simulink model "quadcopter_model"  (R2021a)
settings: Solver=VariableStepAuto  StartTime=0.0  StopTime=500  RelTol=1e-3
values from neighbouring files (symbols this model uses):
  additive_noise = 0    [variables.m]
  initialCondition = [x0 vx0 y0 vy0 z0 vz0 phi0 p0 theta0 q0 psi0 r0]    [variables.m]
  param = [m;Ix;Iy;Iz;l;g]    [variables.m]
libraries: dspsrcs4 x1
settings Model: Creator=fiori  LastModifiedBy=fiori
settings SolverCC: AlgebraicLoopSolver=TrustRegion
settings DebuggingCC: SFMachineParentedDataDiag=warning

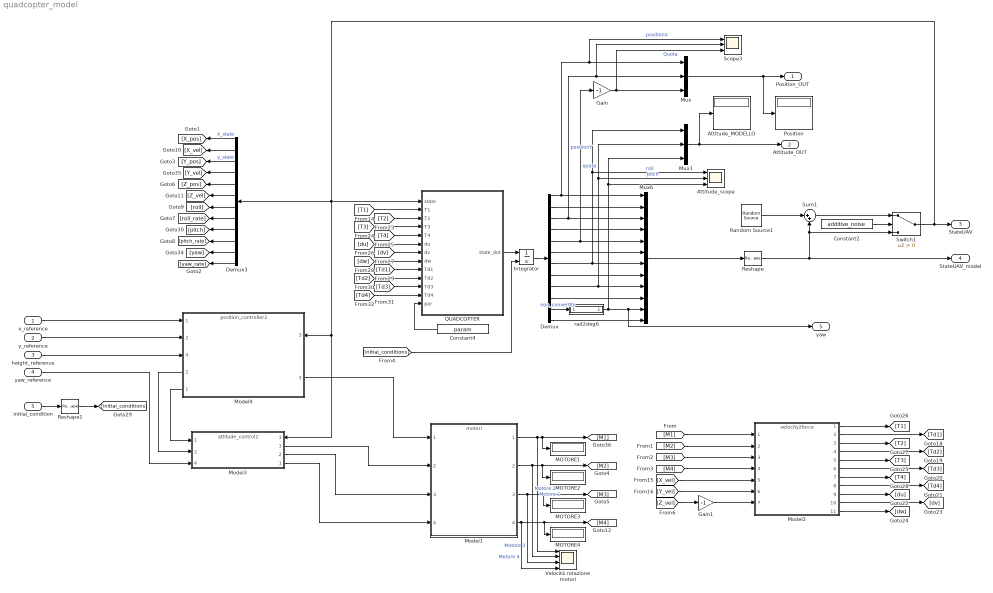
== system quadcopter_model ==
  x_reference : Inport
  y_reference : Inport  Port=2
  height_reference : Inport  Port=3
  yaw_reference : Inport  Port=4
  initial_condition : Inport  Port=5
  Attitude_MODELLO : Display
  Attitude_scope : Scope  NumInputPorts=3
  Constant2 : Constant  Value=additive_noise
  Constant4 : Constant  Value=param
  Demux : Demux  Outputs=12
  Demux3 : Demux  Outputs=12
  Gain : Gain  Gain=-1
  Gain1 : Gain  Gain=-1
  Integrator : Integrator  InitialConditionSource=external  InitialCondition=initialCondition
  MOTORE{1..4} (4 alike) : Display
  Model1 : ModelReference  ModelNameDialog=motori.slx  SimulationMode=Normal  ModelReferenceVersion=1.1
  Model2 : ModelReference  ModelNameDialog=velocity2force.slx  SimulationMode=Normal  ModelReferenceVersion=1.6
  Model3 : ModelReference  ModelNameDialog=attitude_control2.slx  SimulationMode=Normal  ModelReferenceVersion=2.5
      settings: PortSchema="{\"entries\":[{\"content\":{\"sides\":[{\"content\":{\"connectorIds\":[\"In1\",\"In2\",\"In4\"]},\"type\":\"ConnectorPlacement.EquallySpacedRectSide\",\"uuid\":\"61a521c8-5baa-43cc-8c6a-72ed0ccf90cc\"},{\"content\":{\"connectorIds\":[\"In3\",\"Out3\",\"Out2\",\"Out1\"],\"side\":\"RIGHT\"},\"type\":\"ConnectorPlacement.EquallySpacedRectSide\",\"uuid\":\"94cea425-f186-4678-aad1-a22f04fccbca\"},{\"content\":{\"connectorIds\":[],\"side\":\"TOP\"},\"type\":\"ConnectorPlacement.EquallySpacedRectSide\",\"uuid\":\"43df5e5d-9414-4141-a0bf-f7593089cf19\"},{\"content\":{\"connectorIds\":[],\"side\":\"HIDDEN\"},\"type\":\"ConnectorPlacement.EquallySpacedRectSide\",\"uuid\":\"8291e6b4-8c9b-43ee-8ad2-00c7c1575f70\"}]},\"type\":\"ConnectorPlacement.EquallySpacedConnector\",\"uuid\":\"f72a1838-f29b-4d3c-8dc3-12763affa3f1\"}],\"packageUris\":[\"http://schema.mathworks.com/mf0/Connector/R2020b\"],\"version\":\"1.0\"}"
  Model4 : ModelReference  ModelNameDialog=position_controller2.slx  SimulationMode=Normal  ModelReferenceVersion=2.7
      settings: PortSchema="{\"entries\":[{\"content\":{\"sides\":[{\"content\":{\"connectorIds\":[\"In1\",\"In2\",\"In4\",\"Out2\",\"Out1\"]},\"type\":\"ConnectorPlacement.EquallySpacedRectSide\",\"uuid\":\"61a521c8-5baa-43cc-8c6a-72ed0ccf90cc\"},{\"content\":{\"connectorIds\":[\"In3\",\"Out3\"],\"side\":\"RIGHT\"},\"type\":\"ConnectorPlacement.EquallySpacedRectSide\",\"uuid\":\"94cea425-f186-4678-aad1-a22f04fccbca\"},{\"content\":{\"connectorIds\":[],\"side\":\"TOP\"},\"type\":\"ConnectorPlacement.EquallySpacedRectSide\",\"uuid\":\"43df5e5d-9414-4141-a0bf-f7593089cf19\"},{\"content\":{\"connectorIds\":[],\"side\":\"HIDDEN\"},\"type\":\"ConnectorPlacement.EquallySpacedRectSide\",\"uuid\":\"8291e6b4-8c9b-43ee-8ad2-00c7c1575f70\"}]},\"type\":\"ConnectorPlacement.EquallySpacedConnector\",\"uuid\":\"f72a1838-f29b-4d3c-8dc3-12763affa3f1\"}],\"packageUris\":[\"http://schema.mathworks.com/mf0/Connector/R2020b\"],\"version\":\"1.0\"}"
  Mux : Mux  Inputs=3
  Mux1 : Mux  Inputs=3
  Mux6 : Mux  Inputs=12
  Position : Display
  QUADCOPTER : MATLAB Function  TreatAsAtomicUnit=on
  Random Source1 : dspsrcs4/Random Source  SrcType=Gaussian  NormMethod=Ziggurat  CltLength=12  MinVal=0  MaxVal=1  MeanVal=0  VarVal=1e-3  RepMode=Not repeatable  rawSeed=1  IsInherit=off  SampMode=Discrete  SampTime=1  SampFrame=1  DataType=Double  OutComplex=Real  OutputFrames=off
  Reshape : Reshape  OutputDimensionality=Customize  OutputDimensions=[12,1]
  Reshape1 : Reshape  OutputDimensionality=Customize  OutputDimensions=[12,1]
  Scope3 : Scope  NumInputPorts=3
  Sum1 : Sum  Inputs=|++
  Switch1 : Switch  Criteria=u2 > Threshold
  Velocità rotazione motori : Scope  NumInputPorts=4
  rad2deg6 : MATLAB Function  TreatAsAtomicUnit=on
  Position_OUT : Outport
  Attitude_OUT : Outport  Port=2
  StateUAV : Outport  Port=3
  StateUAV_model : Outport  Port=4
  yaw : Outport  Port=5
  wires:
  Demux/3 -> Mux6/3, Scope3/2, Mux/2  "positionY"
  [initial_conditions] -> Integrator/2
  Mux1/1 -> Attitude_MODELLO/1, Attitude_OUT/1
  Demux/12 -> Mux6/12
  Demux/1 -> Mux6/1, Scope3/1, Mux/1  "positionX"
  Demux/8 -> Mux6/8
  Demux/10 -> Mux6/10
  Demux/5 -> Mux6/5, Gain/1  "quota"
  Demux/11 -> rad2deg6/1(angle)  "non_convertito"
  Demux/7 -> Mux6/7, Attitude_scope/1, Mux1/1  "roll"
  Demux/9 -> Mux6/9, Attitude_scope/2, Mux1/2  "pitch"
  height_reference/1 -> Model4/4
  y_reference/1 -> Model4/2
  x_reference/1 -> Model4/1
  Gain/1 -> Scope3/3, Mux/3  "Quota"
  Demux/2 -> Mux6/2
  Demux/4 -> Mux6/4
  Demux/6 -> Mux6/6
  Mux/1 -> Position/1, Position_OUT/1
  rad2deg6/1(angle_rad) -> yaw/1, Mux6/11, Attitude_scope/3, Mux1/3
  Integrator/1 -> Demux/1
  Constant2/1 -> Switch1/2
  Sum1/1 -> Switch1/1
  Random Source1/1 -> Sum1/1
  Demux3/1 -> [X_pos]  "X_stato"
  Demux3/7 -> [roll]
  Demux3/5 -> [Z_pos]
  Demux3/4 -> [Y_vel]
  Demux3/6 -> [Z_vel]
  Demux3/3 -> [Y_pos]  "y_state"
  Demux3/2 -> [X_vel]
  Demux3/9 -> [pitch]
  Demux3/11 -> [yaw]
  Demux3/8 -> [roll_rate]
  Demux3/12 -> [yaw_rate]
  Demux3/10 -> [pitch_rate]
  Switch1/1 -> StateUAV/1, QUADCOPTER/1(state), Model3/3, Model4/3, Demux3/1
  Reshape/1 -> Switch1/3, Sum1/2, StateUAV_model/1
  [T1] -> QUADCOPTER/2(T1)
  [T2] -> QUADCOPTER/3(T2)
  [T3] -> QUADCOPTER/4(T3)
  [T4] -> QUADCOPTER/5(T4)
  [du] -> QUADCOPTER/6(du)
  [dv] -> QUADCOPTER/7(dv)
  [dw] -> QUADCOPTER/8(dw)
  [Td2] -> QUADCOPTER/10(Td2)
  [Td1] -> QUADCOPTER/9(Td1)
  [Td3] -> QUADCOPTER/11(Td3)
  [Td4] -> QUADCOPTER/12(Td4)
  QUADCOPTER/1(state_dot) -> Integrator/1
  Constant4/1 -> QUADCOPTER/13(par)
  Model3/1 -> Model1/4
  Model3/2 -> Model1/3
  Model4/3 -> Model1/1
  Model4/1 -> Model3/1
  Model4/2 -> Model3/2
  Model1/1 -> Velocità rotazione motori/1, MOTORE1/1, [M1]  "Motore 1"
  Model1/2 -> Velocità rotazione motori/2, MOTORE2/1, [M2]  "Motore 2"
  Model1/3 -> Velocità rotazione motori/3, MOTORE3/1, [M3]  "Motore 3"
  Model1/4 -> Velocità rotazione motori/4, MOTORE4/1, [M4]  "Motore 4"
  Model3/3 -> Model1/2
  [M4] -> Model2/4
  [M3] -> Model2/3
  [M2] -> Model2/2
  [M1] -> Model2/1
  [Z_vel] -> Gain1/1
  [Y_vel] -> Model2/6
  [X_vel] -> Model2/5
  Gain1/1 -> Model2/7
  Model2/2 -> [Td1]
  Model2/4 -> [Td2]
  Model2/6 -> [Td3]
  Model2/8 -> [Td4]
  Model2/9 -> [du]
  Model2/10 -> [dv]
  Model2/11 -> [dw]
  Model2/1 -> [T1]
  Model2/3 -> [T2]
  Model2/5 -> [T3]
  Model2/7 -> [T4]
  initial_condition/1 -> Reshape1/1
  Reshape1/1 -> [initial_conditions]
  yaw_reference/1 -> Model3/4
  Mux6/1 -> Reshape/1

== matlab function quadcopter_model/QUADCOPTER ==
  data: state input; state_dot output; T1 input; T2 input; T3 input; T4 input; du input; dv input; dw input; Td1 input; Td2 input; Td3 input; Td4 input; par input
function state_dot = Quadcopter_Dynamics(state,T1,T2,T3,T4,du,dv,dw,Td1,Td2,Td3,Td4,par)
m=par(1);
Ix=par(2);
Iy=par(3);
Iz=par(4);
l=par(5);
g=par(6);

u=state(2);
v=state(4);
z=state(5);
w=state(6);

%ATTITUDE
%ROLL
phi=state(7);
p=state(8);
%PITCH
theta=state(9);
q=state(10);
%YAW
psi=state(11);
r=state(12);

x_dot=u*cos(psi)*cos(theta) - v*cos(phi)*sin(psi) + w*sin(phi)*sin(psi) + w*cos(phi)*cos(psi)*sin(theta) + v*cos(psi)*sin(phi)*sin(theta);
y_dot=v*cos(phi)*cos(psi) - w*cos(psi)*sin(phi) + u*cos(theta)*sin(psi) + w*cos(phi)*sin(psi)*sin(theta) + v*sin(phi)*sin(psi)*sin(theta);
z_dot=w*cos(phi)*cos(theta) - u*sin(theta) + v*cos(theta)*sin(phi);

%Linear accelerations
u_dot = r*v - q*w - g*sin(theta);
v_dot = p*w - r*u + g*cos(theta)*sin(phi);
spinta2= (1/m)*(T1+T2+T3+T4);
if z<-0.01
    w_dot = q*u - p*v + g*cos(phi)*cos(theta) - spinta2; 
else
    w_dot = q*u - p*v - spinta2;
end

phi_dot=(p*cos(theta) + r*cos(phi)*sin(theta) + q*sin(phi)*sin(theta))/cos(theta);
theta_dot=q*cos(phi) - r*sin(phi);
psi_dot=(r*cos(phi) + q*sin(phi))/cos(theta);

p_dot = (l/Ix)*(T2 - T4) - q*r*((Iz-Iy)/(Ix)); 
q_dot = (l/Iy)*(T1 - T3) - p*r*((Ix-Iz)/(Iy));
r_dot = (1/Iz)*(Td2 + Td4 - Td1 - Td3);

u_dot=u_dot - du;
v_dot=v_dot - dv;
w_dot=w_dot - dw;

state_dot = [x_dot, u_dot, y_dot, v_dot, z_dot, w_dot, phi_dot, p_dot, theta_dot, q_dot, psi_dot, r_dot]';

== matlab function quadcopter_model/rad2deg6 ==
  data: angle input; angle_rad output
function angle_rad = fcn(angle)
    angle_rad = angle - 2*pi*floor(angle/(2*pi));
end
